simulink model "testw"  (R2021a)
settings: Solver=VariableStepAuto  StartTime=0.0  StopTime=10.0  RelTol=1e-3
libraries: simulink x1
settings Model: Creator=Aero  LastModifiedBy=Aero

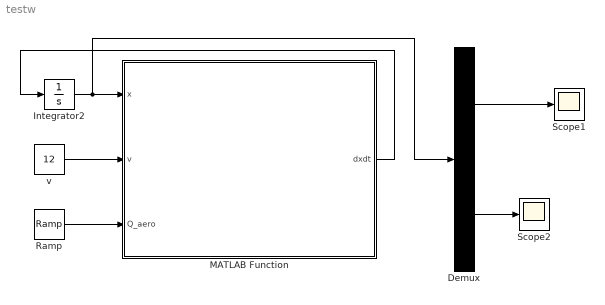
== system testw ==
  Demux : Demux  Outputs=2
  Integrator2 : Integrator  InitialCondition=[1; 20]
  MATLAB Function : MATLAB Function  TreatAsAtomicUnit=on
  Ramp : simulink/Sources/Ramp  slope=0.05  start=0  InitialOutput=0
  Scope1 : Scope
  Scope2 : Scope
  v : Constant  Value=12
  wires:
  Ramp/1 -> MATLAB Function/3(Q_aero)
  v/1 -> MATLAB Function/2(v)
  Integrator2/1 -> Demux/1, MATLAB Function/1(x)
  MATLAB Function/1(dxdt) -> Integrator2/1
  Demux/1 -> Scope1/1
  Demux/2 -> Scope2/1

== matlab function testw/MATLAB Function ==
  data: x input; dxdt output; v input; Q_aero input
function dxdt = fcn(x, v, Q_aero)
    % System parameters
    R = 0.5;      % Resistance (Ohm)
    L = 0.001;    % Inductance (H)
    J_rot = 0.01; % Rotational inertia (kg*m^2)
    K_v = 0.1;    % Speed constant (V*s/rad)
    K_Q = 0.1;    % Torque constant (N*m/A)
    i_0 = 0.5;    % No-load current (A)
    
    % Extract states
    i = x(1);
    omega = x(2);
    
    % Calculate derivatives
    di_dt = (v - omega/K_v - i*R)/L;
    domega_dt = ((i-i_0)/K_Q - Q_aero)/J_rot;
    
    % Return derivative vector
    dxdt = [di_dt; domega_dt];
end
